simulink model "StepResponseSLX"  (R2016a)
settings: Solver=FixedStepDiscrete  StartTime=0.0  StopTime=3.5e-8  FixedStep=5e-13  RelTol=1e-3
values from neighbouring files (symbols this model uses):
  Rg = 1.5    [DPTSpiceMFile.m]    (also in LossCalcModelMFile.m; StepResponse.m)
  Ron = 15    [DPTSpiceMFile.m]    (also in LossCalcModelMFile.m = 20)
  Rs = 0.0433 + 1e-4    (= 0.0434)    [DPTSpiceMFile.m]    (also in LossCalcModelMFile.m = 2.5e-05; StepResponse.m)
  VpulseMax = 7    [DPTSpiceMFile.m]    (also in LossCalcModelMFile.m = 6; StepResponse.m = 6)
  VpulseMin = -3    [DPTSpiceMFile.m]    (also in LossCalcModelMFile.m; StepResponse.m)
libraries: elec_lib x9, nesl_utility x4, fl_lib x3, simulink x1
settings Model: Creator=kkfrk  LastModifiedBy=kkfrk

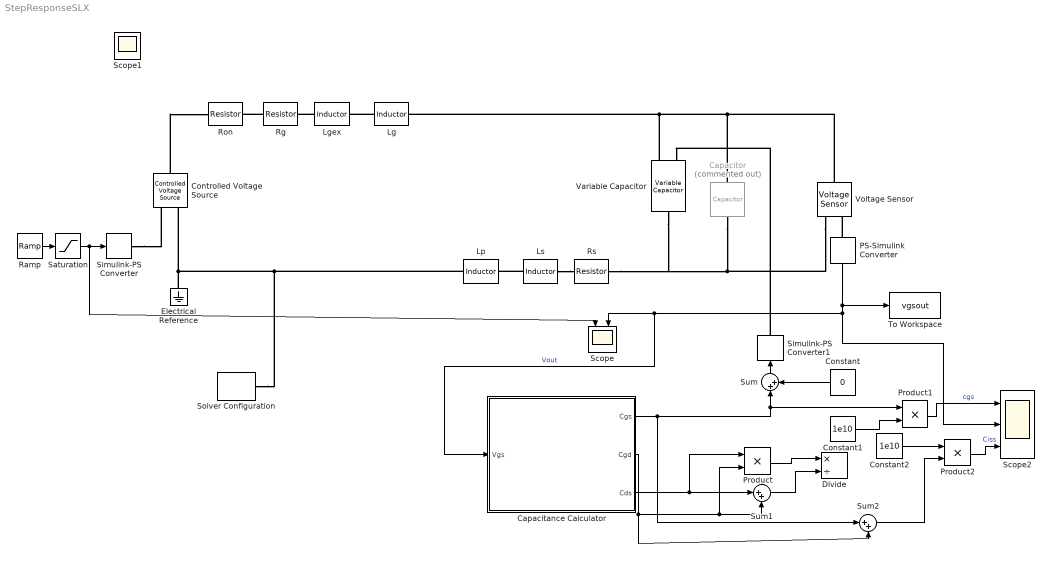
== system StepResponseSLX ==
  Capacitance Calculator : Subsystem
  Capacitor : elec_lib/Passive Devices/Capacitor  Commented=on  enable_table=0  c=Cgd F  Cvec=[ 1e-5 1e-6 ] F  Vvec=[ 0 10 ] V  CV_table_symmetry=1  C_tol=5  enable_C_tol=0  tol_distribution=1  nSigma=4  r=1e-6 Ohm  g=0 1/Ohm  initV=VpulseMin V  enable_operating_limits=0  operating_limit_action=2  max_working_voltage_range=[ -25 25 ] V  power_rating=1 W  enable_faults=0  fault_action=1  Cscale_faulted=100  R_faulted=0.001 Ohm  G_faulted=0 1/Ohm  tau_fault=0.001 s  enable_temporal_fault=0  t_fault=1 s  enable_behavioral_fault=0  max_permissible_voltage_range=[ -100 100 ] V  t_fail_on_voltage=1 s
  Constant : Constant  Value=0
  Constant1 : Constant  Value=1e10
  Constant2 : Constant  Value=1e10
  Controlled Voltage Source : fl_lib/Electrical/Electrical Sources/Controlled Voltage Source
  Divide : Product  Inputs=*/
  Electrical Reference : fl_lib/Electrical/Electrical Elements/Electrical Reference
  Lg : elec_lib/Passive Devices/Inductor  l=Lg H  L_tol=20  enable_L_tol=0  tol_distribution=1  nSigma=4  r=0 Ohm  g=1e-9 1/Ohm  initI=0 A  enable_operating_limits=0  operating_limit_action=2  max_working_current=1 A  power_rating=1 W  enable_faults=0  fault_action=1  lambdaPercent=50  k_faulted=0.9999 Ohm  turnsShort=0  openCct=0  groundShort=0  groundShortG=0 1/Ohm  tau_fault=0.001 s  enable_temporal_fault=0  t_fault=1 s  enable_behavioral_fault=0  max_permissible_voltage=100 V  n_fail_on_voltage=1  max_permissible_current=1 A  t_fail_on_current=1 s
  Lgex : elec_lib/Passive Devices/Inductor  l=Lgex H  L_tol=20  enable_L_tol=0  tol_distribution=1  nSigma=4  r=0 Ohm  g=1e-9 1/Ohm  initI=0 A  enable_operating_limits=0  operating_limit_action=1  max_working_current=1 A  power_rating=1 W  enable_faults=0  fault_action=1  lambdaPercent=50  k_faulted=0.9999 Ohm  turnsShort=0  openCct=0  groundShort=0  groundShortG=0 1/Ohm  tau_fault=0.001 s  enable_temporal_fault=0  t_fault=1 s  enable_behavioral_fault=0  max_permissible_voltage=100 V  n_fail_on_voltage=1  max_permissible_current=1 A  t_fail_on_current=1 s
  Lp : elec_lib/Passive Devices/Inductor  l=Lp H  L_tol=20  enable_L_tol=0  tol_distribution=1  nSigma=4  r=0 Ohm  g=1e-9 1/Ohm  initI=0 A  enable_operating_limits=0  operating_limit_action=2  max_working_current=1 A  power_rating=1 W  enable_faults=0  fault_action=1  lambdaPercent=50  k_faulted=0.9999 Ohm  turnsShort=0  openCct=0  groundShort=0  groundShortG=0 1/Ohm  tau_fault=0.001 s  enable_temporal_fault=0  t_fault=1 s  enable_behavioral_fault=0  max_permissible_voltage=100 V  n_fail_on_voltage=1  max_permissible_current=1 A  t_fail_on_current=1 s
  Ls : elec_lib/Passive Devices/Inductor  l=Ls H  L_tol=20  enable_L_tol=0  tol_distribution=1  nSigma=4  r=0 Ohm  g=1e-9 1/Ohm  initI=0 A  enable_operating_limits=0  operating_limit_action=2  max_working_current=1 A  power_rating=1 W  enable_faults=0  fault_action=1  lambdaPercent=50  k_faulted=0.9999 Ohm  turnsShort=0  openCct=0  groundShort=0  groundShortG=0 1/Ohm  tau_fault=0.001 s  enable_temporal_fault=0  t_fault=1 s  enable_behavioral_fault=0  max_permissible_voltage=100 V  n_fail_on_voltage=1  max_permissible_current=1 A  t_fail_on_current=1 s
  PS-Simulink Converter : nesl_utility/PS-Simulink Converter  PhysicalDomain=network_engine_domain  SubClassName=ps_output  LeftPortType=input  RightPortType=output  PseudoPeriodic=off  Frequencies=[]  Unit=1  AffineConversion=off
  Product : Product
  Product1 : Product
  Product2 : Product
  Ramp : simulink/Sources/Ramp  slope=(VpulseMax-VpulseMin)/1e-9  start=2e-9  X0=VpulseMin
  Rg : elec_lib/Passive Devices/Resistor  R=Rg Ohm  R_tol=5  enable_R_tol=0  tol_distribution=1  nSigma=4  enable_operating_limits=0  operating_limit_action=2  max_working_voltage=100 V  power_rating=1 W  enable_faults=0  fault_action=1  R_faulted=Inf Ohm  enable_temporal_fault=0  t_fault=1 s  enable_behavioral_fault=0  max_permissible_current=1 A  t_fail_on_current=1 s  noise_mode=0  sample_time=0.001 s  repeatability=1  auto_seed=2776703895  user_seed=0  Tdevice=25 degC  alpha=0.00393 1/K  Tmeas=25 degC  thermal_mass=100 J/K  initial_temperature=25 degC  power_derating_T1=70 degC  power_derating_T2=155 degC  operating_temperature_range_vec=[ -50 150 ] degC
  Ron : elec_lib/Passive Devices/Resistor  R=Ron Ohm  R_tol=5  enable_R_tol=0  tol_distribution=1  nSigma=4  enable_operating_limits=0  operating_limit_action=2  max_working_voltage=100 V  power_rating=1 W  enable_faults=0  fault_action=1  R_faulted=Inf Ohm  enable_temporal_fault=0  t_fault=1 s  enable_behavioral_fault=0  max_permissible_current=1 A  t_fail_on_current=1 s  noise_mode=0  sample_time=0.001 s  repeatability=1  auto_seed=3140818123  user_seed=0  Tdevice=25 degC  alpha=0.00393 1/K  Tmeas=25 degC  thermal_mass=100 J/K  initial_temperature=25 degC  power_derating_T1=70 degC  power_derating_T2=155 degC  operating_temperature_range_vec=[ -50 150 ] degC
  Rs : elec_lib/Passive Devices/Resistor  R=Rs Ohm  R_tol=5  enable_R_tol=0  tol_distribution=1  nSigma=4  enable_operating_limits=0  operating_limit_action=2  max_working_voltage=100 V  power_rating=1 W  enable_faults=0  fault_action=1  R_faulted=Inf Ohm  enable_temporal_fault=0  t_fault=1 s  enable_behavioral_fault=0  max_permissible_current=1 A  t_fail_on_current=1 s  noise_mode=0  sample_time=0.001 s  repeatability=1  auto_seed=1967382518  user_seed=0  Tdevice=25 degC  alpha=0.00393 1/K  Tmeas=25 degC  thermal_mass=100 J/K  initial_temperature=25 degC  power_derating_T1=70 degC  power_derating_T2=155 degC  operating_temperature_range_vec=[ -50 150 ] degC
  Saturation : Saturate  UpperLimit=VpulseMax  LowerLimit=VpulseMin
  Scope : Scope  NumInputPorts=2
  Scope2 : Scope  NumInputPorts=3
  Simulink-PS Converter : nesl_utility/Simulink-PS Converter  PhysicalDomain=network_engine_domain  SubClassName=ps_input  LeftPortType=input  RightPortType=output  PseudoPeriodic=off  Frequencies=[]  NoiseDistribution=none  NoiseParameters=[]  Unit=1  AffineConversion=off  InputFiltering=off  SimscapeFilterOrder=1  InputFilterTimeConstant=0.001  UdotUserProvided=1
  Simulink-PS Converter1 : nesl_utility/Simulink-PS Converter  PhysicalDomain=network_engine_domain  SubClassName=ps_input  LeftPortType=input  RightPortType=output  PseudoPeriodic=off  Frequencies=[]  NoiseDistribution=none  NoiseParameters=[]  Unit=1  AffineConversion=off  InputFiltering=off  SimscapeFilterOrder=1  InputFilterTimeConstant=0.001  UdotUserProvided=1
  Solver Configuration : nesl_utility/Solver Configuration  PhysicalDomain=network_engine_domain  SubClassName=solver  LeftPortType=input  RightPortType=generic  Accelerate=off  Tones=[]  Harmonics=[]  SimulateNoise=off  Profile=off  UseLocalSampling=off  EnableSwitchedLinearOptims=on  FrequencyDomain=off  UseCCode=off  RelTol=0.001  AbsTol=1e-06  MinStep=1e-09  ToWorkspace=off  RevertToSquareIcSolve=off  NumHomotopyIterations=100  PhasorMode=off  PhasorModeNumHarmonics=1  OverrideAbsTol=off  DoDC=off  ResidualTolerance=1e-09  UseLocalSolver=on  LocalSolverChoice=NE_BACKWARD_EULER_ADVANCER  LocalSolverSampleTime=5e-13  DoFixedCost=on  MaxNonlinIter=3  MaxModeIter=2  LinearAlgebra=Sparse  DelaysMemoryBudget=1024  AutomaticFiltering=on  FilteringTimeConstant=0.001
  Sum : Sum  Inputs=|++
  Sum1 : Sum  Inputs=|++
  Sum2 : Sum  Inputs=|++
  To Workspace : ToWorkspace  VariableName=vgsout  SampleTime=-1
  Variable Capacitor : elec_lib/Passive Devices/Variable Capacitor  prm=2  Cmin=1e-17 F  r=1e-6 Ohm  v0=VpulseMin V  q0=0 c
  Voltage Sensor : fl_lib/Electrical/Electrical Sensors/Voltage Sensor
  Scope1 : Scope
  wires:
  PS-Simulink Converter/1 -> Scope2/2, Capacitance Calculator/1(Vgs), Scope/2, To Workspace/1  "Vout"
  Capacitance Calculator/2(Cgd) -> Sum2/2, Product/2, Sum1/2
  Capacitance Calculator/3(Cds) -> Product/1, Sum1/1
  Product/1 -> Divide/1
  Sum1/1 -> Divide/2
  Sum/1 -> Simulink-PS Converter1/1
  Capacitance Calculator/1(Cgs) -> Sum2/1, Product1/1, Sum/1
  Constant/1 -> Sum/2
  Ramp/1 -> Saturation/1
  Saturation/1 -> Scope/1, Simulink-PS Converter/1
  Product1/1 -> Scope2/1  "cgs"
  Constant1/1 -> Product1/2
  Product2/1 -> Scope2/3  "Ciss"
  Constant2/1 -> Product2/1
  Sum2/1 -> Product2/2
  connections:
  Simulink-PS Converter/RConn1 -- Controlled Voltage Source/RConn1
  Voltage Sensor/LConn1 -- Capacitor/LConn1 -- Lg/RConn1 -- Variable Capacitor/LConn2
  Voltage Sensor/RConn2 -- Rs/LConn1 -- Variable Capacitor/RConn1 -- Capacitor/RConn1
  PS-Simulink Converter/LConn1 -- Voltage Sensor/RConn1
  Simulink-PS Converter1/RConn1 -- Variable Capacitor/LConn1
  Rg/LConn1 -- Ron/RConn1
  Lgex/LConn1 -- Rg/RConn1
  Lg/LConn1 -- Lgex/RConn1
  Controlled Voltage Source/LConn1 -- Ron/LConn1
  Ls/LConn1 -- Rs/RConn1
  Ls/RConn1 -- Lp/LConn1
  Lp/RConn1 -- Solver Configuration/RConn1 -- Electrical Reference/LConn1 -- Controlled Voltage Source/RConn2

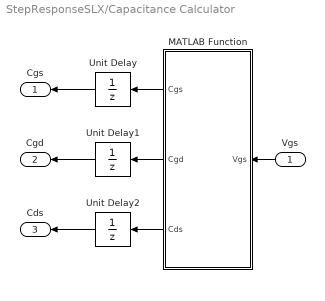
== system StepResponseSLX/Capacitance Calculator ==
  Vgs : Inport
  MATLAB Function : MATLAB Function  TreatAsAtomicUnit=on
  Unit Delay : UnitDelay  InitialCondition=258e-12  SampleTime=-1
  Unit Delay1 : UnitDelay  InitialCondition=63e-12  SampleTime=-1
  Unit Delay2 : UnitDelay  InitialCondition=2e-12  SampleTime=-1
  Cgs : Outport
  Cgd : Outport  Port=2
  Cds : Outport  Port=3
  wires:
  Vgs/1 -> MATLAB Function/1(Vgs)
  MATLAB Function/1(Cgs) -> Unit Delay/1
  MATLAB Function/2(Cgd) -> Unit Delay1/1
  MATLAB Function/3(Cds) -> Unit Delay2/1
  Unit Delay/1 -> Cgs/1
  Unit Delay1/1 -> Cgd/1
  Unit Delay2/1 -> Cds/1

== matlab function StepResponseSLX/Capacitance Calculator/MATLAB Function ==
  data: Vgs input; Cgs output; Cgd output; Cds output
function [Cgs,Cgd,Cds]= fcn(Vgs)
%#codegen
Vds = 400;% - (Vgs+3)*400/9;
%% Crss calculation
       a1 =   2.519e+14;
       b1 =      -345.7;
       c1 =       63.76;
       a2 =       27.99;
       b2 =       12.86;
       c2 =       18.29;
       a3 =       8.666;
       b3 =       33.93;
       c3 =       9.161;
       a4 =       1.502;
       b4 =       125.5;
       c4 =       121.9;
       a5 =      0.6563;
       b5 =         500;
       c5 =       34.57;
       a6 =        1.98;
       b6 =       408.2;
       c6 =       134.7;
Crss = a1.*exp(-((Vds-b1)./c1).^2) + a2.*exp(-((Vds-b2)./c2).^2) + a3*exp(-((Vds-b3)./c3).^2)...
   + a4.*exp(-((Vds-b4)./c4).^2) +a5.*exp(-((Vds-b5)./c5).^2) +a6.*exp(-((Vds-b6)./c6).^2);
Crss = Crss*1e-12;
%% Ciss Calculation
%        a1 =        1167;
%        b1 =      -115.8;
%        c1 =       60.96;
%        a2 =       269.7;
%        b2 =       -5402;
%        c2 =   4.243e+04;
%        a3 =        3.61;
%        b3 =       238.5;
%        c3 =       2.507;
%        a4 =       1.036;
%        b4 =       175.8;
%        c4 =       16.81;
%        a5 =       1.571;
%        b5 =         263;
%        c5 =       3.586;
%        a6 =      -1.174;
%        b6 =       238.2;
%        c6 =       25.85;
       a1 =        267.6;
       b1 =      2.007;
       c1 =       0.4734;
       a2 =       240.1;
       b2 =       3.049;
       c2 =      1.104;
       a3 =        -1336;
       b3 =       7.803;
       c3 =       9.331;
       a4 =       -250.6;
       b4 =       7.082;
       c4 =       1.715;
       a5 =       -2352;
       b5 =         11.25;
       c5 =       3.184;
       a6 =      8.572e13;
       b6 =       340.6;
       c6 =       67.72;
Ciss = a1.*exp(-((Vgs-b1)./c1).^2) + a2.*exp(-((Vgs-b2)./c2).^2) + a3*exp(-((Vgs-b3)./c3).^2)...
   + a4.*exp(-((Vgs-b4)./c4).^2) +a5.*exp(-((Vgs-b5)./c5).^2) +a6.*exp(-((Vgs-b6)./c6).^2);
Ciss = Ciss*1e-12;
%% Coss Calculation
       a1 =         328;
       b1 =       -8.43;
       c1 =       30.26;
       a2 =       115.8;
       b2 =        42.2;
       c2 =       7.341;
       a3 =       45.83;
       b3 =       59.01;
       c3 =       6.099;
       a4 =       183.1;
       b4 =        28.6;
       c4 =       16.39;
       a5 =       69.29;
       b5 =       154.4;
       c5 =        1511;
       a6 =       125.6;
       b6 =       22.68;
       c6 =       119.6;
Coss = a1.*exp(-((Vds-b1)./c1).^2) + a2.*exp(-((Vds-b2)./c2).^2) + a3*exp(-((Vds-b3)./c3).^2)...
   + a4.*exp(-((Vds-b4)./c4).^2) +a5.*exp(-((Vds-b5)./c5).^2) +a6.*exp(-((Vds-b6)./c6).^2);
Coss = Coss*1e-12;
%% Outputs
Cgs = Ciss - Crss;
Cds = Coss - Crss;
Cgd = Crss;
